simulink model "washingMachine"  (R2024b)
settings: Solver=VariableStepAuto  StartTime=0.0  StopTime=inf  RelTol=1e-3
settings Model: Creator=user  LastModifiedBy=user

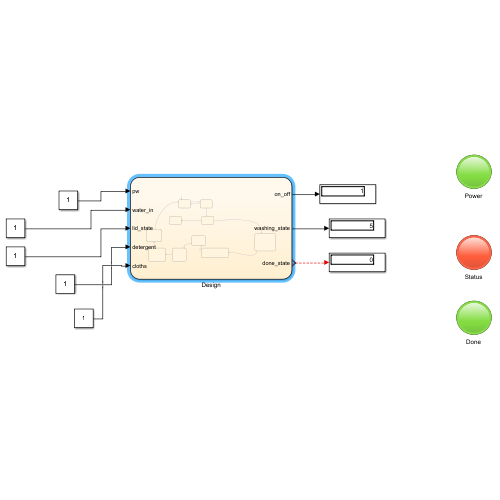
[thumbnail: Simulink's stored preview of the top-level diagram]
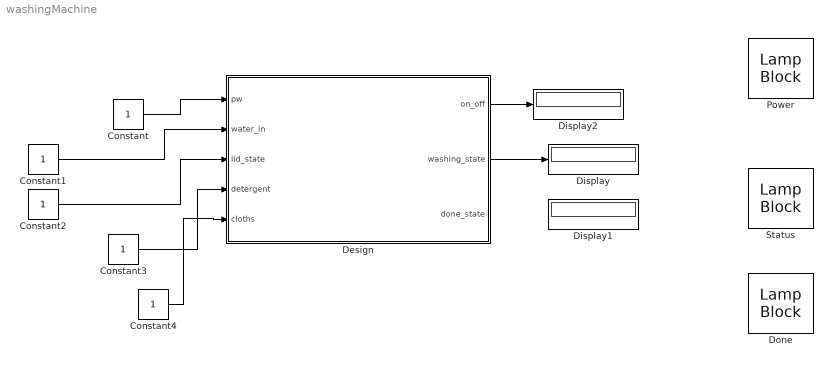
== system washingMachine ==
  Constant{,1..4} (5 alike) : Constant
  Design : Stateflow chart  TreatAsAtomicUnit=on
  Display : Display
  Display1 : Display
  Display2 : Display
  Done : LampBlock  LabelPosition=Hide
  Power : LampBlock  LabelPosition=Hide
  Status : LampBlock  LabelPosition=Hide
  wires:
  Constant1/1 -> Design/2(water_in)
  Constant/1 -> Design/1(pw)
  Constant2/1 -> Design/3(lid_state)
  Constant3/1 -> Design/4(detergent)
  Constant4/1 -> Design/5(cloths)
  Design/2(washing_state) -> Display/1
  ? -> Display1/1
  Design/1(on_off) -> Display2/1

== stateflow chart washingMachine/Design ==
  state power_off
    on_off=0;
  state power_on
    on_off=1;
  state water_low
    water=0;
  state water_state
  state done
    done_state=1;
    washing_state=0;
  state water_high
    water=1;
    lid=1;
    cloths_state=1;
    detergent_state=1;
  state valve
    entry:
    water=0;
    exit:
    water=1;
  state spin
    washing_state=5;
    exit:
    washing_state=6;
  state rinse
    entry:
    washing_state=3;
    exit:
    washing_state=4;
  state wash
    entry:
    washing_state=1;
    exit:
    washing_state=2;
  (default) -> power_off
  done -> power_off : [pw==0]
  power_off -> power_on : [pw==1]
  power_on -> power_off [order 1] : [pw==0]
  power_on -> water_state [order 2]
  water_state -> water_high [order 1] : [lid_state==1&&...
      | cloths==1&&detergent==1&&water_in==1]
  water_state -> water_low [order 2] : [water_in==0]
  spin -> done : after(30,sec)
  valve -> rinse
  wash -> valve : after(30,sec)
  water_high -> wash
  rinse -> spin : after(30,sec)
  data: pw input; on_off output; water_in input; lid_state input; detergent input; lid local; detergent_state local; cloths_state local; cloths input; washing_state output; water local; done_state output
